simulink model "massSpringMDL"  (R2014a)
settings: Solver=ode45  StartTime=0.0  StopTime=TSIM  RelTol=1e-3
values from neighbouring files (symbols this model uses):
  c = 1    [massSpring.m]
  d = 10    [bookEx.m]    (also in massSpring.m = 5)
  k = k1+k2    [carsus.m]    (also in massSpring.m = 1)
  m = 1    [massSpring.m]
  x1_0 = 100    [bookEx.m]    (also in massSpring.m = -1)
  x2_0 = -100    [bookEx.m]    (also in massSpring.m = -5)
  x3_0 = 1    [bookEx.m]    (also in massSpring.m)
  x4_0 = 1    [massSpring.m]
undefined symbols (not defined in the file or in its folder): Klqr
settings Model: Creator=sqn4594  LastModifiedBy=sqn4594

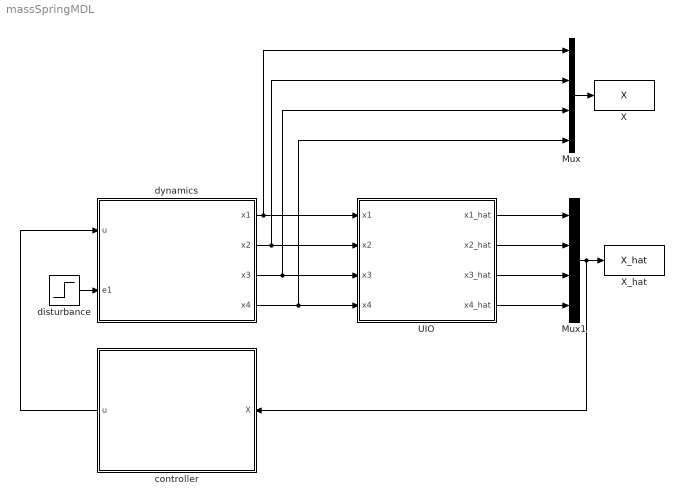
== system massSpringMDL ==
  Mux : Mux
  Mux1 : Mux
  UIO : Subsystem
  X : ToWorkspace  VariableName=X  SampleTime=-1
  X_hat : ToWorkspace  VariableName=X_hat  SampleTime=-1
  controller : Subsystem
  disturbance : Step  Time=d  After=2  SampleTime=0
  dynamics : Subsystem
  wires:
  Mux1/1 -> controller/1(X), X_hat/1
  disturbance/1 -> dynamics/2(e1)
  controller/1(u) -> dynamics/1(u)
  dynamics/1(x1) -> UIO/1(x1), Mux/1
  dynamics/4(x4) -> Mux/4, UIO/4(x4)
  dynamics/2("x2 ") -> UIO/2(x2), Mux/2
  dynamics/3(x3) -> UIO/3(x3), Mux/3
  UIO/4(x4_hat) -> Mux1/4
  UIO/2(x2_hat) -> Mux1/2
  UIO/3(x3_hat) -> Mux1/3
  UIO/1(x1_hat) -> Mux1/1
  Mux/1 -> X/1

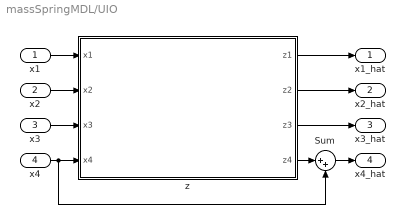
== system massSpringMDL/UIO ==
  x1 : Inport
  x2 : Inport  Port=2
  x3 : Inport  Port=3
  x4 : Inport  Port=4
  Sum : Sum  Inputs=|++
  z : Subsystem
  x1_hat : Outport
  x2_hat : Outport  Port=2
  x3_hat : Outport  Port=3
  x4_hat : Outport  Port=4
  wires:
  x1/1 -> z/1(x1)
  x2/1 -> z/2(x2)
  x4/1 -> Sum/2, z/4(x4)
  x3/1 -> z/3(x3)
  z/1(z1) -> x1_hat/1
  z/2(z2) -> x2_hat/1
  z/3(z3) -> x3_hat/1
  z/4(z4) -> Sum/1
  Sum/1 -> x4_hat/1

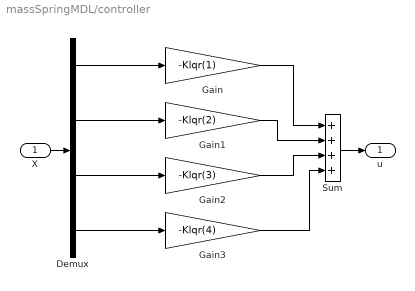
== system massSpringMDL/controller ==
  X : Inport
  Demux : Demux
  Gain : Gain  Gain=-Klqr(1)
  Gain1 : Gain  Gain=-Klqr(2)
  Gain2 : Gain  Gain=-Klqr(3)
  Gain3 : Gain  Gain=-Klqr(4)
  Sum : Sum  Inputs=++++
  u : Outport
  wires:
  X/1 -> Demux/1
  Demux/1 -> Gain/1
  Demux/2 -> Gain1/1
  Demux/3 -> Gain2/1
  Demux/4 -> Gain3/1
  Sum/1 -> u/1
  Gain/1 -> Sum/1
  Gain1/1 -> Sum/2
  Gain2/1 -> Sum/3
  Gain3/1 -> Sum/4

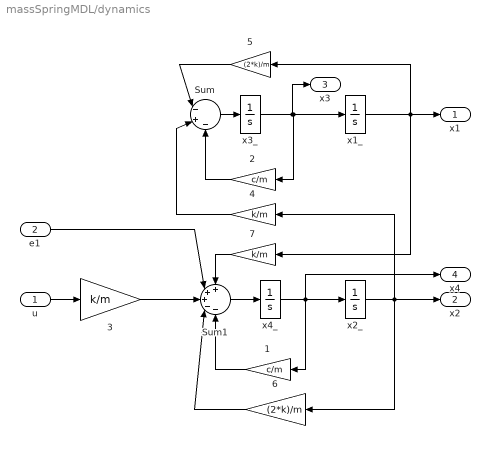
== system massSpringMDL/dynamics ==
  u : Inport
  e1 : Inport  Port=2
  "  1" : Gain  Gain=c/m
  "  2" : Gain  Gain=c/m
  "  3" : Gain  Gain=k/m
  "  4" : Gain  Gain=k/m
  "  5" : Gain  Gain=(2*k)/m
  "  6" : Gain  Gain=(2*k)/m
  "  7" : Gain  Gain=k/m
  Sum : Sum  Inputs=|-+-
  Sum1 : Sum  Inputs=+++--
  x1_ : Integrator  InitialCondition=x1_0
  x2_ : Integrator  InitialCondition=x2_0
  x3_ : Integrator  InitialCondition=x3_0
  x4_ : Integrator  InitialCondition=x4_0
  x1 : Outport
  "x2 " : Outport  Port=2
  x3 : Outport  Port=3
  x4 : Outport  Port=4
  wires:
  u/1 -> "  3"/1
  Sum/1 -> x3_/1
  x3_/1 -> "  2"/1, x1_/1, x3/1
  Sum1/1 -> x4_/1
  "  3"/1 -> Sum1/3
  x1_/1 -> "  7"/1, "  5"/1, x1/1
  x2_/1 -> "  6"/1, "  4"/1, "x2 "/1
  x4_/1 -> "  1"/1, x4/1, x2_/1
  "  2"/1 -> Sum/3
  "  5"/1 -> Sum/1
  "  1"/1 -> Sum1/5
  "  6"/1 -> Sum1/4
  "  7"/1 -> Sum1/1
  "  4"/1 -> Sum/2
  e1/1 -> Sum1/2

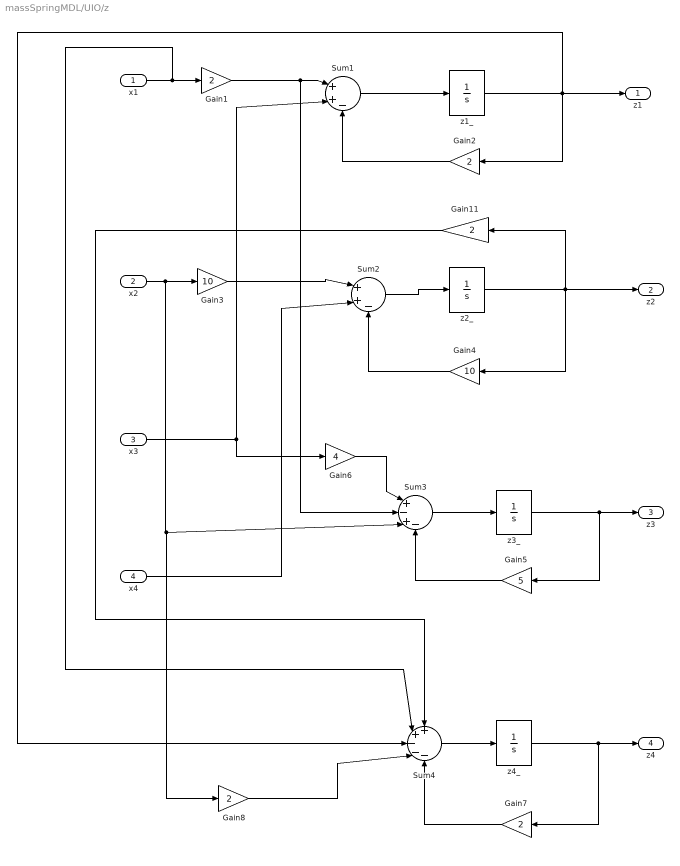
== system massSpringMDL/UIO/z ==
  x1 : Inport
  x2 : Inport  Port=2
  x3 : Inport  Port=3
  x4 : Inport  Port=4
  Gain{1..2,7..8,11} (5 alike) : Gain  Gain=2
  Gain3 : Gain  Gain=10
  Gain4 : Gain  Gain=10
  Gain5 : Gain  Gain=5
  Gain6 : Gain  Gain=4
  Sum1 : Sum  Inputs=|++-
  Sum2 : Sum  Inputs=|++-
  Sum3 : Sum  Inputs=|+-+-
  Sum4 : Sum  Inputs=++---
  z1_ : Integrator
  z2_ : Integrator
  z3_ : Integrator
  z4_ : Integrator
  z1 : Outport
  z2 : Outport  Port=2
  z3 : Outport  Port=3
  z4 : Outport  Port=4
  wires:
  x1/1 -> Sum4/2, Gain1/1
  Gain1/1 -> Sum3/2, Sum1/1
  Sum1/1 -> z1_/1
  z1_/1 -> Gain2/1, Sum4/3, z1/1
  Gain2/1 -> Sum1/3
  x3/1 -> Sum1/2, Gain6/1
  x2/1 -> Gain8/1, Sum3/3, Gain3/1
  Gain3/1 -> Sum2/1
  x4/1 -> Sum2/2
  Sum2/1 -> z2_/1
  z2_/1 -> Gain11/1, z2/1, Gain4/1
  Gain4/1 -> Sum2/3
  z3_/1 -> z3/1, Gain5/1
  Sum3/1 -> z3_/1
  Gain5/1 -> Sum3/4
  Gain6/1 -> Sum3/1
  z4_/1 -> z4/1, Gain7/1
  Sum4/1 -> z4_/1
  Gain7/1 -> Sum4/5
  Gain8/1 -> Sum4/4
  Gain11/1 -> Sum4/1
